simulink model "Testrunde"  (R2025b)
settings: Solver=VariableStepAuto  StartTime=0.0  StopTime=10.0  RelTol=1e-3
settings Model: Creator=henni  LastModifiedBy=henni

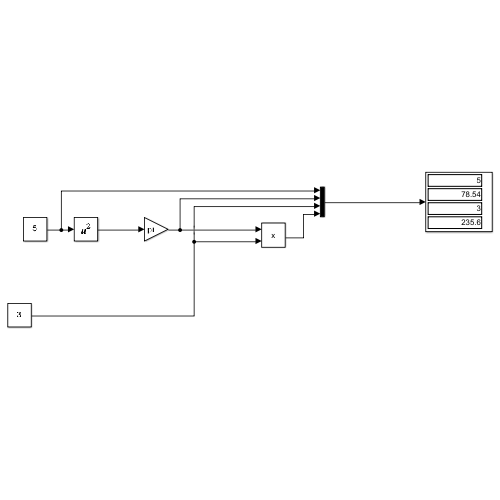
[thumbnail: Simulink's stored preview of the top-level diagram]
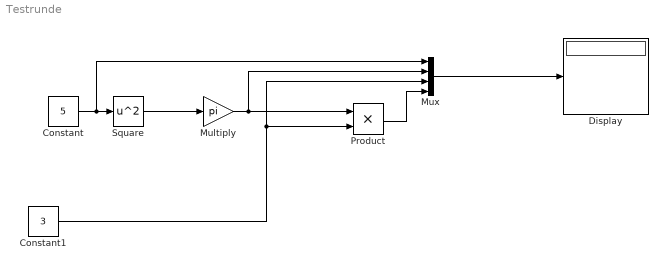
== system Testrunde ==
  Constant : Constant  Value=5
  Constant1 : Constant  Value=3
  Display : Display
      settings: Decimation=2
  Multiply : Gain  Gain=pi
  Mux : Mux
  Product : Product
  Square : Math  Operator=square
  wires:
  Constant/1 -> Mux/1, Square/1
  Square/1 -> Multiply/1
  Mux/1 -> Display/1
  Constant1/1 -> Product/2, Mux/3
  Multiply/1 -> Product/1, Mux/2
  Product/1 -> Mux/4
